simulink model "band_1_test"  (Simulink 7.8)
settings: Solver=ode45  StartTime=0.0  StopTime=10.0  RelTol=1e-3
undefined symbols (not defined in the file or in its folder): Fs, get
libraries: dsparch4 x4, dspsrcs4 x1, dspsnks4 x1
settings Model: Creator=svenhoffmann  LastModifiedBy=josef  ExtModeAutoUpdateStatusClock=off
settings DataIOCC: SignalLoggingName=sigsOut
settings OptimizationCC: InitFltsAndDblsToZero=on
settings DebuggingCC: SaveWithParameterizedLinksMsg=none  SignalResolutionControl=TryResolveAllWithWarning  SolverPrmCheckMsg=none  MultiTaskDSMMsg=warning  MultiTaskCondExecSysMsg=none  FcnCallInpInsideContextMsg=Use local settings  StrictBusMsg=None
settings HardwareCC: TargetUnknown=on
settings RTWCC: IncludeERTFirstTime=on
settings GRTTargetCC: TargetFcnLib=ansi_tfl_tmw.mat

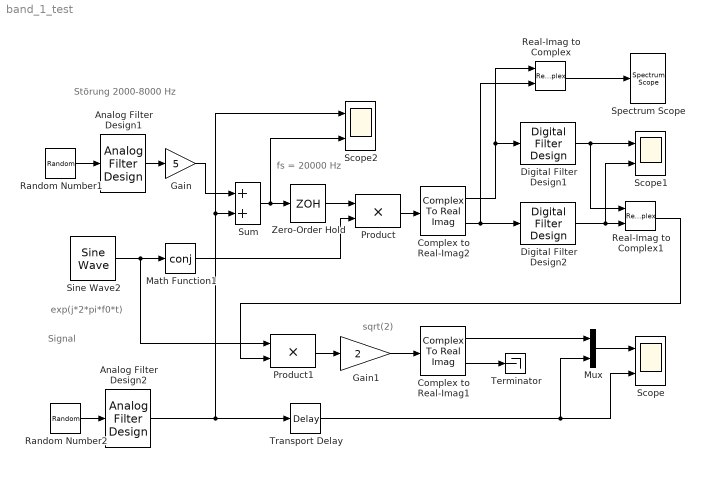
== system band_1_test ==
  note: sqrt(2)
  note: Signal
  note: exp(j*2*pi*f0*t)
  note: Störung
      | 2000-8000 Hz
  note: fs =
      | 20000 Hz
  Analog Filter Design1 : dsparch4/Analog Filter Design  method=Chebyshev I  filttype=Bandpass  N=8  Wlo=2*pi*2000  Whi=2*pi*8000  Rp=2  Rs=40
  Analog Filter Design2 : dsparch4/Analog Filter Design  method=Chebyshev I  filttype=Bandpass  N=8  Wlo=2*pi*990  Whi=2*pi*1020  Rp=2  Rs=40
  Complex to Real-Imag1 : ComplexToRealImag
  Complex to Real-Imag2 : ComplexToRealImag
  Digital Filter Design1 : dsparch4/Digital Filter Design  mwdsp_browser_bugfix_var=off
  Digital Filter Design2 : dsparch4/Digital Filter Design  mwdsp_browser_bugfix_var=off
  Gain : Gain  Gain=5  SaturateOnIntegerOverflow=on  OutDataTypeStr=Inherit: Same as input  ParamDataTypeStr=Inherit: Same as input
  Gain1 : Gain  Gain=2  SaturateOnIntegerOverflow=on  OutDataTypeStr=Inherit: Same as input  ParamDataTypeStr=Inherit: Same as input
  Math Function1 : Math  Operator=conj  SaturateOnIntegerOverflow=on
  Mux : Mux  Inputs=2
  Product : Product  SaturateOnIntegerOverflow=on  OutDataTypeStr=Inherit: Same as first input
  Product1 : Product  SaturateOnIntegerOverflow=on  OutDataTypeStr=Inherit: Same as first input
  Random Number1 : RandomNumber  SampleTime=0
  Random Number2 : RandomNumber  Seed=174536  SampleTime=0
  Real-Imag to Complex : RealImagToComplex
  Real-Imag to Complex1 : RealImagToComplex
  Scope : Scope  NumInputPorts=2
      settings: YMin=-1.25~-1  YMax=1.25~1  MaxDataPoints=500000
  Scope1 : Scope  NumInputPorts=2
      settings: YMin=-1~-0.75  YMax=1~0.75  MaxDataPoints=500000
  Scope2 : Scope  NumInputPorts=2
      settings: YMin=-2.5~-2.5  YMax=3~3  SaveName=ScopeData2  MaxDataPoints=500000
  Sine Wave2 : dspsrcs4/Sine Wave  Amplitude=1  Frequency=1000  Phase=0  SampleMode=Discrete  OutComplex=Complex  CompMethod=Table lookup  TableSize=Speed  SampleTime=1/20000  SamplesPerFrame=1  ResetState=Restart at time zero  dataType=double  wordLen=16  udDataType=sfix(16)  fracBitsMode=Best precision  numFracBits=15  OutDataTypeStr=double  LastOutDataTypeStr=double
      settings: additionalParams=on
  Spectrum Scope : dspsnks4/Spectrum Scope  ScopeProperties=off  Domain=Frequency  HorizSpan=1  UseBuffer=on  BufferSize=256  Overlap=64  TreatMby1Signals=M channels  inpFftLenInherit=off  FFTlength=128  numAvg=10  DisplayProperties=off  AxisGrid=on  Memory=off  FrameNumber=on  AxisLegend=off  AxisZoom=off  OpenScopeAtSimStart=on  OpenScopeImmediately=off  FigPos=get(0,'defaultfigureposition')  AxisProperties=on  XUnits=Hertz  XRange=[-Fs/2...Fs/2]  XDisplay=0  InheritXIncr=on  XIncr=1.  XLabel=Samples  XLimit=Auto  YUnits=dB  XMax=1  XMin=0  YLabel=Magnitude, dB  LineProperties=off  wintypeSpecScope=Hann  RsSpecScope=50  betaSpecScope=5  winsampSpecScope=Periodic  XAxisParamsVer=6.8  isFrameUpgraded=on
      settings: YMin=-68.3560619370471  YMax=20.509723098933
  Sum : Sum  SaturateOnIntegerOverflow=on
  Terminator : Terminator
  Transport Delay : TransportDelay  DelayTime=0
  Zero-Order Hold : ZeroOrderHold  SampleTime=1/20000
  wires:
  Analog Filter Design2/1 -> Transport Delay/1, Sum/2, Scope2/1
  Random Number1/1 -> Analog Filter Design1/1
  Analog Filter Design1/1 -> Gain/1
  Gain/1 -> Sum/1
  Sum/1 -> Zero-Order Hold/1, Scope2/2
  Zero-Order Hold/1 -> Product/1
  Sine Wave2/1 -> Math Function1/1, Product1/1
  Mux/1 -> Scope/1
  Transport Delay/1 -> Mux/2, Scope/2
  Product1/1 -> Gain1/1
  Gain1/1 -> Complex to Real-Imag1/1
  Product/1 -> Complex to Real-Imag2/1
  Complex to Real-Imag2/1 -> Digital Filter Design1/1, Real-Imag to Complex/1
  Complex to Real-Imag2/2 -> Digital Filter Design2/1, Real-Imag to Complex/2
  Digital Filter Design1/1 -> Real-Imag to Complex1/1, Scope1/1
  Digital Filter Design2/1 -> Scope1/2, Real-Imag to Complex1/2
  Real-Imag to Complex1/1 -> Product1/2
  Complex to Real-Imag1/1 -> Mux/1
  Math Function1/1 -> Product/2
  Real-Imag to Complex/1 -> Spectrum Scope/1
  Random Number2/1 -> Analog Filter Design2/1
  Complex to Real-Imag1/2 -> Terminator/1
